simulink model "adaptativeControl"  (R2023b)
settings: Solver=VariableStepAuto  StartTime=0.0  StopTime=time(end)  FixedStep=10e-17  RelTol=1e-3
undefined symbols (not defined in the file or in its folder): DiscIntNeverNeededParam
libraries: simulink x1
settings Model: Creator=v4pal  LastModifiedBy=v4pal

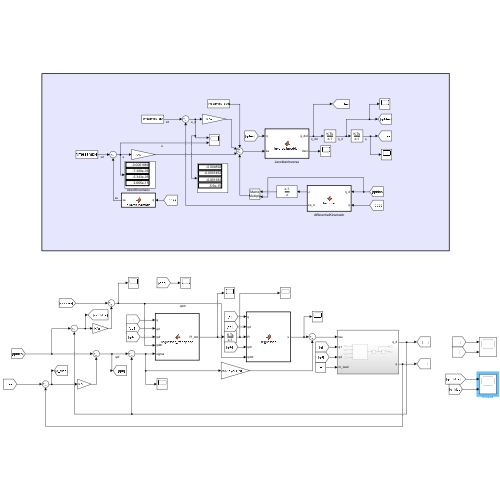
[thumbnail: Simulink's stored preview of the top-level diagram]
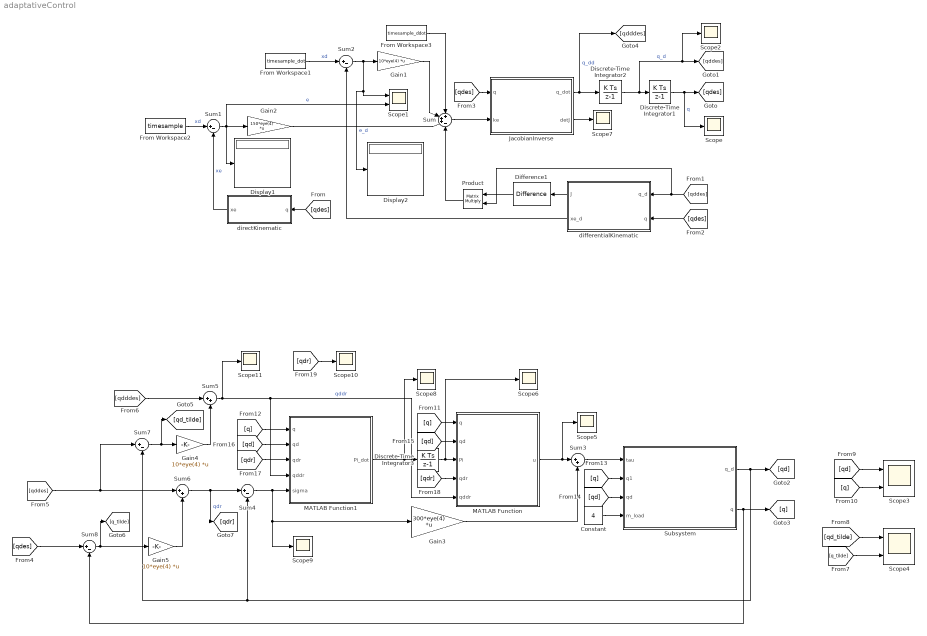
== system adaptativeControl ==
  Constant : Constant  Value=4
  Difference1 : simulink/Discrete/Difference  ICPrevInput=0.0  OutMin=[]  OutMax=[]  OutDataType=fixdt(1, 16)  OutScaling=2^-10  DoSatur=off
  Discrete-Time Integrator1 : DiscreteIntegrator  InitialCondition=[-1.1781; 0.7851; -0.5000; 0.3930]  SampleTime=0.001  ICPrevOutput=DiscIntNeverNeededParam  ICPrevScaledInput=DiscIntNeverNeededParam
  Discrete-Time Integrator2 : DiscreteIntegrator  InitialCondition=[0; 0; 0; 0]  SampleTime=0.001  ICPrevOutput=DiscIntNeverNeededParam  ICPrevScaledInput=DiscIntNeverNeededParam
  Discrete-Time Integrator3 : DiscreteIntegrator  InitialCondition=[1.2500, 20.0000, 5.0000, 1.2500, 10.0000, 4, 4.000, 4.0000, 1.0000, 0.0100, 0.0100, 0.0050, 0.0010, 0.0001, 0.0001, 0.0100, 0.0050]'  SampleTime=0.001  ICPrevOutput=DiscIntNeverNeededParam  ICPrevScaledInput=DiscIntNeverNeededParam
  Display1 : Display
  Display2 : Display
  From Workspace1 : FromWorkspace  VariableName=timesample_dot
  From Workspace2 : FromWorkspace  VariableName=timesample
  From Workspace3 : FromWorkspace  VariableName=timesample_ddot
  Gain1 : Gain  Gain=10*eye(4)  Multiplication=Matrix(K*u)
  Gain2 : Gain  Gain=150*eye(4)  Multiplication=Matrix(K*u)
  Gain3 : Gain  Gain=300*eye(4)  Multiplication=Matrix(K*u)
  Gain4 : Gain  Gain=10*eye(4)  Multiplication=Matrix(K*u)
  Gain5 : Gain  Gain=10*eye(4)  Multiplication=Matrix(K*u)
  JacobianInverse : MATLAB Function  TreatAsAtomicUnit=on
  MATLAB Function : MATLAB Function  TreatAsAtomicUnit=on
  MATLAB Function1 : MATLAB Function  TreatAsAtomicUnit=on
  Product : Product  Multiplication=Matrix(*)
  Scope{,2,5..11} (9 alike) : Scope
  Scope1 : Scope  NumInputPorts=2
  Scope3 : Scope  NumInputPorts=2
  Scope4 : Scope  NumInputPorts=2
  Subsystem : Subsystem
  Sum : Sum  Inputs=+++-
  Sum{1..2,4,7..8} (5 alike) : Sum  Inputs=|+-
  Sum3 : Sum  Inputs=|++
  Sum5 : Sum  Inputs=|++
  Sum6 : Sum  Inputs=|++
  differentialKinematic : MATLAB Function  TreatAsAtomicUnit=on
  directKinematic : MATLAB Function  TreatAsAtomicUnit=on
  wires:
  Gain1/1 -> Sum/2
  Difference1/1 -> Product/1
  From Workspace1/1 -> Sum2/1  "xd"
  [qddes] -> Product/2, differentialKinematic/1(q_d)
  [qdes] -> differentialKinematic/2(q)
  differentialKinematic/1(J) -> Difference1/1
  From Workspace3/1 -> Sum/1
  Product/1 -> Sum/4
  Discrete-Time Integrator1/1 -> Scope/1, [qdes]  "q"
  Sum2/1 -> Display2/1, Scope1/1, Gain1/1  "e_d"
  Discrete-Time Integrator2/1 -> Scope2/1, [qddes], Discrete-Time Integrator1/1  "q_d"
  differentialKinematic/2(xe_d) -> Sum2/2
  JacobianInverse/2(detJ) -> Scope7/1
  [qdes] -> directKinematic/1(q)
  directKinematic/1(xe) -> Sum1/2  "xe"
  Gain2/1 -> Sum/3
  Sum1/1 -> Scope1/2, Display1/1, Gain2/1  "e"
  [qdes] -> JacobianInverse/1(q)
  JacobianInverse/1(q_dot) -> [qdddes], Discrete-Time Integrator2/1  "q_dd"
  Sum/1 -> JacobianInverse/2(ke)
  From Workspace2/1 -> Sum1/1  "xd"
  [q] -> Scope3/2
  [qd] -> Scope3/1
  Sum3/1 -> Subsystem/1(tau)
  Gain3/1 -> Sum3/2
  Discrete-Time Integrator3/1 -> MATLAB Function/3(Pi), Scope6/1
  Sum4/1 -> MATLAB Function1/5(sigma), Scope9/1, Gain3/1
  Gain4/1 -> Sum5/2
  Gain5/1 -> Sum6/2
  Sum6/1 -> [qdr], Sum4/1  "qdr"
  Subsystem/1(q_d) -> [qd], Sum7/2, Sum4/2
  Sum8/1 -> Gain5/1, [q_tilde]
  Sum7/1 -> [qd_tilde], Gain4/1
  Sum5/1 -> Scope11/1, MATLAB Function1/4(qddr), MATLAB Function/5(qddr)  "qddr"
  Subsystem/2(q) -> [q], Sum8/2
  Constant/1 -> Subsystem/4(m_load)
  [qd_tilde] -> Scope4/1
  [q_tilde] -> Scope4/2
  [q] -> MATLAB Function/1(q)
  [q] -> MATLAB Function1/1(q)
  [q] -> Subsystem/2(q1)
  [qd] -> Subsystem/3(qd)
  [qd] -> MATLAB Function/2(qd)
  [qd] -> MATLAB Function1/2(qd)
  [qdr] -> MATLAB Function1/3(qdr)
  [qdr] -> MATLAB Function/4(qdr)
  MATLAB Function/1(u) -> Scope5/1, Sum3/1
  [qdr] -> Scope10/1
  MATLAB Function1/1(Pi_dot) -> Scope8/1, Discrete-Time Integrator3/1
  [qddes] -> Sum6/1, Sum7/1
  [qdddes] -> Sum5/1
  [qdes] -> Sum8/1

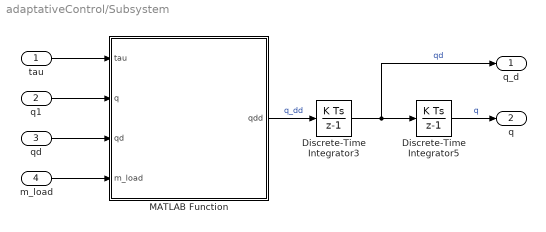
== system adaptativeControl/Subsystem ==
  tau : Inport
  q1 : Inport  Port=2
  qd : Inport  Port=3
  m_load : Inport  Port=4
  Discrete-Time Integrator3 : DiscreteIntegrator  InitialCondition=[0; 0; 0; 0]  SampleTime=0.001  ICPrevOutput=DiscIntNeverNeededParam  ICPrevScaledInput=DiscIntNeverNeededParam
  Discrete-Time Integrator5 : DiscreteIntegrator  InitialCondition=[-1.1781; 0.7851; -0.5000; 0.3930]  SampleTime=0.001  ICPrevOutput=DiscIntNeverNeededParam  ICPrevScaledInput=DiscIntNeverNeededParam
  MATLAB Function : MATLAB Function  TreatAsAtomicUnit=on
  q_d : Outport
  q : Outport  Port=2
  wires:
  Discrete-Time Integrator5/1 -> q/1  "q"
  Discrete-Time Integrator3/1 -> q_d/1, Discrete-Time Integrator5/1  "qd"
  m_load/1 -> MATLAB Function/4(m_load)
  MATLAB Function/1(qdd) -> Discrete-Time Integrator3/1  "q_dd"
  qd/1 -> MATLAB Function/3(qd)
  q1/1 -> MATLAB Function/2(q)
  tau/1 -> MATLAB Function/1(tau)

== matlab function adaptativeControl/differentialKinematic ==
  data: q_d input; J output; q input; xe_d output
function [J, xe_d] = Jacobian(q_d, q)

    % Init the SCARA manipulator parameters
    a1 = .5; a2 = .5;
    theta1 = q(1,:); theta2 = q(2,:);
    
    %% Geometric Jacobian Matrix
    J_a = [-a1*sin(theta1) - a2*sin(theta1 + theta2), - a2*sin(theta1 + theta2), 0, 0;
        a1*cos(theta1) + a2*cos(theta1 + theta2), a2*cos(theta1 + theta2), 0, 0;
        0, 0, -1, 0;
        1, 1, 0, -1;];

    % Vx = Jx1 * qd1 + Jx2 * qd2 +Jx3 * qd3;
    % Vy = Jy1 * qd1 + Jy2 * qd2 +Jy3 * qd3;
    % Vz = Jz1 * qd1 + Jz2 * qd2 +Jz3 * qd3;
    
    %J = J_a(1:3,1:3);
    J = J_a;

    %% Calculation of xe_dot
    xe_d = J * q_d;

end

== matlab function adaptativeControl/directKinematic ==
  data: q input; xe output
function xe = directKinematic(q)
    
    %% Init the SCARA manipulator parameters and Joint variables
    a1 = .5; a2 = .5; d0 = 1;
    theta1 = q(1,:); theta2 = q(2,:); d3 = q(3,:); theta4 = q(4,:);

    %% Forward Kinematics link for the SCARA
    k = [a1*cos(theta1) + a2*cos(theta1 + theta2);
        a1*sin(theta1) + a2*sin(theta1 + theta2);
        d0 - d3;
        theta1 + theta2 - theta4;];

    xe = k;

end

== matlab function adaptativeControl/MATLAB Function1 ==
  data: q input; Pi_dot output; qd input; qdr input; qddr input; sigma input
function Pi_dot = regressor_transpose(q,qd,qdr,qddr,sigma)


q1 = q(1,:);
q2 = q(2,:);
q3 = q(3,:);
q4 = q(4,:);
qd1 = qd(1,:);
qd2 = qd(2,:);
qd3 = qd(3,:);
qd4 = qd(4,:);
qdr1 = qdr(1,:);
qdr2 = qdr(2,:);
qdr3 = qdr(3,:);
qdr4 = qdr(4,:);
qddr1 = qddr(1,:);
qddr2 = qddr(2,:);
qddr3 = qddr(3,:);
qddr4 = qddr(4,:);

a1 = 0.5;
a2 = 0.5;

ml1 = 20;
ml2 = 20;
ml3 = 10;
m_load = 4;
Il1 = 4;
Il2 = 4;
Il4 = 1;
Im1 = 0.01;
Im2 = 0.01;
Im3 = 0.005;
Im4 = 0.001;
l1 = 0.25;
l2 = 0.25;
kr1 = 1;
kr2 = 1;
kr3 = 50;
kr4 = 20;
Fm1 =  0.00005;
Fm2 =  0.00005;
Fm3 = 0.01;
Fm4 = 0.005;
Pi_0 = [ml1*l1^2, ml2 , ml2*l2 , ml2*l2^2, ml3, Il1, Il2, Il4, Im1, Im2, Im3, Im4, Fm1, Fm2, Fm3, Fm4]';

Y = [qddr1, qddr1*a1^2 + 2*l2*qddr1*cos(q2)*a1, a1*qddr2*cos(q2) - a1*qd1*qdr2*sin(q2) - a1*qd2*qdr1*sin(q2) - a1*qd2*qdr2*sin(q2), qddr1 + qddr2, a1^2*qddr1 + a2^2*qddr1 + a2^2*qddr2 + 2*a1*a2*qddr1*cos(q2) + a1*a2*qddr2*cos(q2) - a1*a2*qd1*qdr2*sin(q2) - a1*a2*qd2*qdr1*sin(q2) - a1*a2*qd2*qdr2*sin(q2), a1^2*qddr1 + a2^2*qddr1 + a2^2*qddr2 + 2*a1*a2*qddr1*cos(q2) + a1*a2*qddr2*cos(q2) - a1*a2*qd1*qdr2*sin(q2) - a1*a2*qd2*qdr1*sin(q2) - a1*a2*qd2*qdr2*sin(q2), qddr1, qddr1 + qddr2, qddr1 + qddr2 - qddr4, kr1^2*qddr1,       qddr1 + kr2*qddr2,           qddr1 + qddr2 + kr3*qddr3,           qddr1 + qddr2 - kr4*qddr4, kr1^2*qdr1,          0,          0,      0;
     0,                                  0,                                             a1*qddr1*cos(q2) + a1*qd1*qdr1*sin(q2), qddr1 + qddr2,                                                                                        a2^2*qddr1 + a2^2*qddr2 + a1*a2*qddr1*cos(q2) + a1*a2*qd1*qdr1*sin(q2),                                                                                        a2^2*qddr1 + a2^2*qddr2 + a1*a2*qddr1*cos(q2) + a1*a2*qd1*qdr1*sin(q2),     0, qddr1 + qddr2, qddr1 + qddr2 - qddr4,           0, qddr2*kr2^2 + qddr1*kr2,           qddr1 + qddr2 + kr3*qddr3,           qddr1 + qddr2 - kr4*qddr4,          0, kr2^2*qdr2,          0,          0;
     0,                                  0,                                                                                  0,             0,                                                                                                                                                qddr3 - 9.8100,                                                                                                                                                qddr3 - 9.8100,     0,             0,                     0,           0,                       0, kr3*qddr1 + kr3*qddr2 + kr3^2*qddr3,                                   0,          0,          0, kr3^2*qdr3,          0;
     0,                                  0,                                                                                  0,             0,                                                                                                                                                             0,                                                                                                                                                             0,     0,             0, qddr4 - qddr2 - qddr1,           0,                       0,                                   0, kr4^2*qddr4 - kr4*qddr2 - kr4*qddr1,          0,          0,          0, kr4^2*qdr4];


K_PI = 50000*eye(17);
% K_PI(6,6) = 60;
% K_PI(12,12) = 4500;
% K_PI(13,13) = 1000;
% K_PI(16,16) = 1000;
Pi_dot = inv(K_PI)*(Y')*sigma;

end

== matlab function adaptativeControl/JacobianInverse ==
  data: q input; ke input; q_dot output; detJ output
function [q_dot, detJ] = inverseJacobian(q, ke) % q = [theta1; theta2]

    % Init the SCARA manipulator parameters
    a1 = .5; a2 = .5;

    theta1 = q(1,:); theta2 = q(2,:);
    %% Geometric Jacobian Matrix
    J = [-a1*sin(theta1) - a2*sin(theta1 + theta2), - a2*sin(theta1 + theta2), 0, 0;
        a1*cos(theta1) + a2*cos(theta1 + theta2), a2*cos(theta1 + theta2), 0, 0;
        0, 0, -1, 0;
        1, 1, 0, -1;];

    % Vx = Jx1 * qd1 + Jx2 * qd2 +Jx3 * qd3;
    % Vy = Jy1 * qd1 + Jy2 * qd2 +Jy3 * qd3;
    % Vz = Jz1 * qd1 + Jz2 * qd2 +Jz3 * qd3;
    
    %J = J(1:3,1:3);
    
    detJ = det(J);
    % Calculate the inverse of the Jacobian matrix
    J_inv = inv(J);

    % Calculate joint velocities
    q_dot = J_inv * ke;

end

== matlab function adaptativeControl/Subsystem/MATLAB Function ==
  data: tau input; q input; qdd output; qd input; m_load input
function qdd = dir_dyn(tau,q,qd,m_load)

q1 = q(1,:);
q2 = q(2,:);
q3 = q(3,:);
q4 = q(4,:);
qd1 = qd(1,:);
qd2 = qd(2,:);

%% parametri
a1 = 0.5;
a2 = 0.5;
d0 = 1;

delta = 0.1;

ml1 = 20;
ml2 = 20;
ml3 = 10;
Il1 = 4;
Il2 = 4;
Il4 = 1;
Im1 = 0.01;
Im2 = 0.01;
Im3 = 0.005;
Im4 = 0.001;
l1 = 0.25;
l2 = 0.25;
kr1 = 1;
kr2 = 1;
kr3 = 50;
kr4 = 20;
Fm1 =  0.00005;
Fm2 =  0.00005;
Fm3 = 0.01;
Fm4 = 0.005;

% Uncertainty
% ml1 = ml1 + delta*ml1; ml2 = ml2 + delta*ml2; ml3 = ml3 + delta*ml3;
% Il1 = Il1 + delta*Il1; Il2 = Il2 + delta*Il2; Il4 = Il4 + delta*Il4;
% l1 = l1 + delta*l1; l2 = l2 + delta*l2;
% Fm1 = Fm1 + delta*Fm1;


%% calcolo p pl z
p0 = [0 ; 0 ; d0];
p1 = [a1*cos(q1) ; a1*sin(q1) ; d0];
p2 = [a1*cos(q1) + a2*cos(q1+q2) ; a1*sin(q1) + a2*sin(q1+q2) ; d0];
p3 = p2 - [0 ; 0 ; q3];
p4 = p3;
pl1 = [l1*cos(q1) ; l1*sin(q1) ; d0];
pl2 = [a1*cos(q1) + l2*cos(q1+q2) ; a1*sin(q1) + l2*sin(q1+q2) ; d0];
pl3 = p3; % ????
pl4 = p4; % 
z0 = [0 0 1]';
z1 = [0 0 1]';
z2 = [0 0 -1]';
z3 = [0 0 -1]';

%% calcolo JPl JOl JOm
JP_l1 = [cross(z0,pl1-p0) zeros(3,3)];
JP_l2 = [cross(z0,pl2-p0) cross(z1,pl2-p1) zeros(3,2)];
JP_l3 = [cross(z0,pl3-p0) cross(z1,pl3-p1) z2 zeros(3,1)]; 
JP_l4 = [cross(z0,pl4-p0) cross(z1,pl4-p1) z2 cross(z3,pl4-p3)]; %m4=mload

JO_l1 = [z0 zeros(3,3)];
JO_l2 = [z0 z1 zeros(3,2)];
%JO_l3 = [z0 z1 zeros(3,2)]; Il3=0
JO_l4 = [z0 z1 zeros(3,1) z3];

%assumo che zm1=z0, zm2=z1, zm3=-z2, zm4=z3-->si trova sul giunto
JO_m1 = JO_l1;
JO_m1(:,1) = kr1*z0;
JO_m2 = JO_l2;  
JO_m2(:,2) = kr2*z1;
JO_m3 = [z0 z1 zeros(3,2)]; 
JO_m3(:,3) = kr3*z2;
JO_m4 = JO_l4;
JO_m4(:,4) = kr4*z3;

%% Matrice d'Inerzia B (eq 7.32)
B1 = ml1*(JP_l1'*JP_l1) + Il1*(JO_l1'*JO_l1) + Im1*(JO_m1'*JO_m1) ; 
B2 = ml2*(JP_l2'*JP_l2) + Il2*(JO_l2'*JO_l2) + Im2*(JO_m2'*JO_m2) ; 
B3 = ml3*(JP_l3'*JP_l3) + 0 + Im3*(JO_m3'*JO_m3) ; %Il3=0
B4 = m_load*(JP_l4'*JP_l4) + Il4*(JO_l4'*JO_l4) + Im4*(JO_m4'*JO_m4) ; 
B = B1 + B2 + B3 + B4;

%% Contributo di gravità sull'iesimo link.(Formula 7.39)
g0 = [0 0 -9.81]';
g1 = - (ml1*g0'*JP_l1(:,1) + ml2*g0'*JP_l2(:,1) + ml3*g0'*JP_l3(:,1) + m_load*g0'*JP_l4(:,1));
g2 = - (ml1*g0'*JP_l1(:,2) + ml2*g0'*JP_l2(:,2) + ml3*g0'*JP_l3(:,2) + m_load*g0'*JP_l4(:,2));
g3 = - (ml1*g0'*JP_l1(:,3) + ml2*g0'*JP_l2(:,3) + ml3*g0'*JP_l3(:,3) + m_load*g0'*JP_l4(:,3));
g4 = - (ml1*g0'*JP_l1(:,4) + ml2*g0'*JP_l2(:,4) + ml3*g0'*JP_l3(:,4) + m_load*g0'*JP_l4(:,4));
g = [g1 g2 g3 g4]';

%% Contributo di accelerazione C
C = [-a1*qd2*sin(q2)*(a2*m_load + a2*ml3 + l2*ml2), -a1*sin(q2)*(qd1 + qd2)*(a2*m_load + a2*ml3 + l2*ml2), 0, 0;
      a1*qd1*sin(q2)*(a2*m_load + a2*ml3 + l2*ml2),  0, 0, 0;
      0, 0, 0, 0;
      0, 0, 0, 0]; 

%% Attrito viscoso al manipolatore
Fv = diag([kr1^2*Fm1 kr2^2*Fm2 kr3^2*Fm3 kr4^2*Fm4]);

%% Calcolo solo l'accelerazione dato che velox e pos si ottengono integrando
qdd = inv(B)*(tau - C*qd -Fv*qd -g);

end

== matlab function adaptativeControl/MATLAB Function ==
  data: q input; u output; qd input; Pi input; qdr input; qddr input
function u= regressor(q,qd,Pi,qdr,qddr)

q1 = q(1,:);
q2 = q(2,:);
q3 = q(3,:);
q4 = q(4,:);
qd1 = qd(1,:);
qd2 = qd(2,:);
qd3 = qd(3,:);
qd4 = qd(4,:);
qdr1 = qdr(1,:);
qdr2 = qdr(2,:);
qdr3 = qdr(3,:);
qdr4 = qdr(4,:);
qddr1 = qddr(1,:);
qddr2 = qddr(2,:);
qddr3 = qddr(3,:);
qddr4 = qddr(4,:);
a1 = 0.5;
a2 = 0.5;

ml1 = 20;
ml2 = 20;
ml3 = 10;
m_load = 4;
Il1 = 4;
Il2 = 4;
Il4 = 1;
Im1 = 0.01;
Im2 = 0.01;
Im3 = 0.005;
Im4 = 0.001;
l1 = 0.25;
l2 = 0.25;
kr1 = 1;
kr2 = 1;
kr3 = 50;
kr4 = 20;
Fm1 =  0.00005;
Fm2 =  0.00005;
Fm3 = 0.01;
Fm4 = 0.005;
Pi_0 = [ml1*l1^2, ml2 , ml2*l2 , ml2*l2^2, ml3, Il1, Il2, Il4, Im1, Im2, Im3, Im4, Fm1, Fm2, Fm3, Fm4]';

Y = [qddr1, qddr1*a1^2 + 2*l2*qddr1*cos(q2)*a1, a1*qddr2*cos(q2) - a1*qd1*qdr2*sin(q2) - a1*qd2*qdr1*sin(q2) - a1*qd2*qdr2*sin(q2), qddr1 + qddr2, a1^2*qddr1 + a2^2*qddr1 + a2^2*qddr2 + 2*a1*a2*qddr1*cos(q2) + a1*a2*qddr2*cos(q2) - a1*a2*qd1*qdr2*sin(q2) - a1*a2*qd2*qdr1*sin(q2) - a1*a2*qd2*qdr2*sin(q2), a1^2*qddr1 + a2^2*qddr1 + a2^2*qddr2 + 2*a1*a2*qddr1*cos(q2) + a1*a2*qddr2*cos(q2) - a1*a2*qd1*qdr2*sin(q2) - a1*a2*qd2*qdr1*sin(q2) - a1*a2*qd2*qdr2*sin(q2), qddr1, qddr1 + qddr2, qddr1 + qddr2 - qddr4, kr1^2*qddr1,       qddr1 + kr2*qddr2,           qddr1 + qddr2 + kr3*qddr3,           qddr1 + qddr2 - kr4*qddr4, kr1^2*qdr1,          0,          0,      0;
     0,                                  0,                                             a1*qddr1*cos(q2) + a1*qd1*qdr1*sin(q2), qddr1 + qddr2,                                                                                        a2^2*qddr1 + a2^2*qddr2 + a1*a2*qddr1*cos(q2) + a1*a2*qd1*qdr1*sin(q2),                                                                                        a2^2*qddr1 + a2^2*qddr2 + a1*a2*qddr1*cos(q2) + a1*a2*qd1*qdr1*sin(q2),     0, qddr1 + qddr2, qddr1 + qddr2 - qddr4,           0, qddr2*kr2^2 + qddr1*kr2,           qddr1 + qddr2 + kr3*qddr3,           qddr1 + qddr2 - kr4*qddr4,          0, kr2^2*qdr2,          0,          0;
     0,                                  0,                                                                                  0,             0,                                                                                                                                                qddr3 - 9.8100,                                                                                                                                                qddr3 - 9.8100,     0,             0,                     0,           0,                       0, kr3*qddr1 + kr3*qddr2 + kr3^2*qddr3,                                   0,          0,          0, kr3^2*qdr3,          0;
     0,                                  0,                                                                                  0,             0,                                                                                                                                                             0,                                                                                                                                                             0,     0,             0, qddr4 - qddr2 - qddr1,           0,                       0,                                   0, kr4^2*qddr4 - kr4*qddr2 - kr4*qddr1,          0,          0,          0, kr4^2*qdr4];
    
u = Y*Pi;
end
